simulink model "Lift_Dragforces"  (R2020a)
settings: Solver=VariableStepAuto  StartTime=0.0  StopTime=6  RelTol=1e-3
model workspace (MAT data in the model file):
  T = Simulink.Parameter
  T.Value = [0; 0; 23.07; 17.74; 13.42; 9.93; 7.08; 4.74; 4.8; 3.17; 1.78; 0.59; -0.44; -1.34; -2.13; -2.83; -3.46; -4.02; -4.52; -4.98; -5.39; -4.77; -5.12; -5.43; -5.73]
  T.DataType = 'auto'
  T.Dimensions = [25 1]
  Tw = Simulink.Parameter
  Tw.Value = [0; 0; 24.07; 18.74; 14.42; 10.93; 8.08; 5.74; 5.8; 4.17; 2.78; 1.59; 0.56; -0.34; -1.13; -1.83; -2.46; -3.02; -3.52; -3.98; -4.39; -3.77; -4.12; -4.43; -4.73]
  Tw.DataType = 'auto'
  Tw.Dimensions = [25 1]
  a = Simulink.Parameter
  a.Value = [0.289798575; 0.30459674; 0.314300855; 0.320590761; 0.324695185; 0.327419595; 0.329266982; 0.330547514; 0.331453787; 0.332107409; 0.3325868; 0.332943702; 0.333213067; 0.333419111; 0.333579107; 0.333705864; 0.333809448; 0.333898539; 0.333981756; 0.334069415; 0.334176808; 0.334332409; 0.334606222; 0.335273105; 0.335273105]
  a.DataType = 'auto'
  a.Dimensions = [25 1]
  ad = Simulink.Parameter
  ad.Value = [1.515241086; 0.637108512; 0.353415361; 0.222386755; 0.151082935; 0.108245808; 0.080683396; 0.062013288; 0.048845254; 0.039248859; 0.032063134; 0.026557986; 0.022256717; 0.018837814; 0.016078029; 0.013817996; 0.011940578; 0.010356505; 0.008993998; 0.007789833; 0.006678523; 0.005571335; 0.004290268; 0.002196383; 0.002196383]
  ad.DataType = 'auto'
  ad.Dimensions = [25 1]
  adp5 = Simulink.Parameter
  adp5.Value = [0; 0; 0.161386935; 0.100936667; 0.068015045; 0.048298399; 0.035668845; 0.027176718; 0.026154004; 0.021248319; 0.017584933; 0.014773712; 0.012576934; 0.010833186; 0.009428602; 0.008287644; 0.007359433; 0.006598956; 0.005984102; 0.005511002; 0.005178535; 0.004044009; 0.004168658; 0.004977863; 0.004977863]
  adp5.DataType = 'auto'
  adp5.Dimensions = [25 1]
  ap5 = Simulink.Parameter
  ap5.Value = [0; 0; 0.197308672; 0.193419158; 0.19060639; 0.188320167; 0.186408424; 0.184780447; 0.18622744; 0.185210871; 0.184412939; 0.183708715; 0.183133563; 0.182715678; 0.182454669; 0.182442554; 0.182866993; 0.183770944; 0.185493747; 0.188781814; 0.194498145; 0.176650898; 0.195168855; 0.240212713; 0.240212713]
  ap5.DataType = 'auto'
  ap5.Dimensions = [25 1]
  c = Simulink.Parameter
  c.Value = [3.65 4.43 4.56 4.36 4.03 3.68 3.35 3.05 2.79 2.56 2.37 2.19 2.04 1.91 1.79 1.68 1.59 1.5 1.43 1.36 1.29 1.24 1.18 1.14 1.09]
  c.DataType = 'auto'
  c.Dimensions = [1 25]
  r = Simulink.Parameter
  r.Value = [1.8; 3.6; 5.4; 7.2; 9; 10.8; 12.6; 14.4; 16.2; 18; 19.8; 21.6; 23.4; 25.2; 27; 28.8; 30.6; 32.4; 34.2; 36; 37.8; 39.6; 41.4; 43.2; 45]
  r.DataType = 'auto'
  r.Dimensions = [25 1]
  wind_speed = [3 5]
libraries: dspsrcs4 x1
settings Model: Creator=Dimple  LastModifiedBy=Dimple
settings SolverCC: AlgebraicLoopSolver=LineSearch

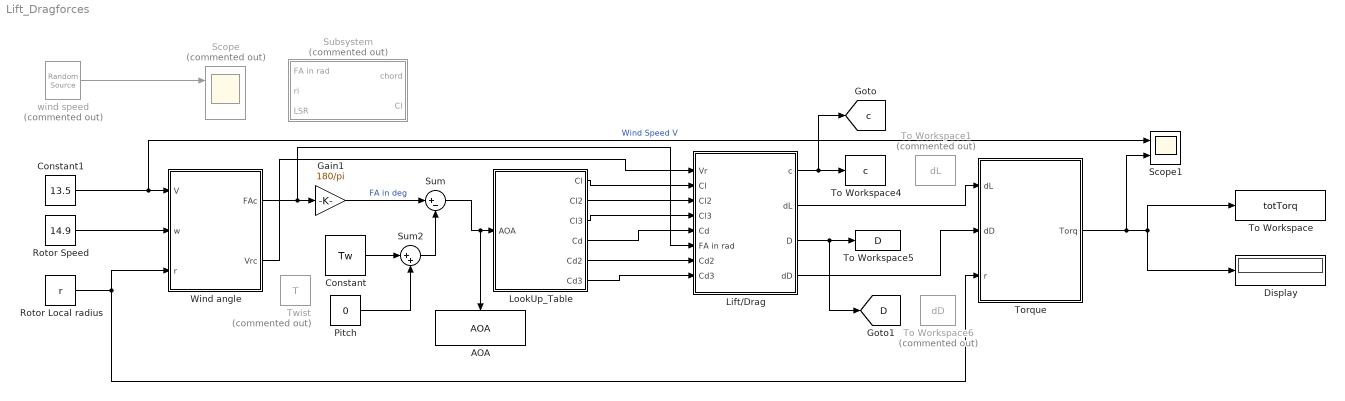
== system Lift_Dragforces ==
  AOA : ToWorkspace  VariableName=AOA  SampleTime=-1
      settings: Save2DSignal=2-D array (concatenate along first dimension)
  Constant : Constant  Value=Tw  VectorParams1D=off  SampleTime=-1
  Constant1 : Constant  Value=13.5
  Display : Display
  Gain1 : Gain  Gain=180/pi
  Lift/Drag : Subsystem
  LookUp_Table : Subsystem
  Pitch : Constant  Value=0
  Rotor Local radius : Constant  Value=r
  Rotor Speed : Constant  Value=14.9  VectorParams1D=off
  Scope : Scope  Commented=on  NumInputPorts=2
  Scope1 : Scope  NumInputPorts=2
  Subsystem : Subsystem  Commented=on
  Sum : Sum  Inputs=|+-
  Sum2 : Sum  Inputs=|++
  To Workspace : ToWorkspace  VariableName=totTorq  SampleTime=-1
      settings: Save2DSignal=2-D array (concatenate along first dimension)
  To Workspace1 : ToWorkspace  Commented=on  VariableName=dL  SampleTime=-1
      settings: Save2DSignal=2-D array (concatenate along first dimension)
  To Workspace4 : ToWorkspace  VariableName=c  SampleTime=-1
      settings: Save2DSignal=2-D array (concatenate along first dimension)
  To Workspace5 : ToWorkspace  VariableName=D  SampleTime=-1
      settings: Save2DSignal=2-D array (concatenate along first dimension)
  To Workspace6 : ToWorkspace  Commented=on  VariableName=dD  SampleTime=-1
      settings: Save2DSignal=2-D array (concatenate along first dimension)
  Torque : Subsystem
  Twist : Constant  Commented=on  Value=T
  Wind angle : Subsystem
  wind speed : dspsrcs4/Random Source  Commented=on  SrcType=Gaussian  NormMethod=Ziggurat  CltLength=12  MinVal=0  MaxVal=1  MeanVal=16  VarVal=2  RepMode=Not repeatable  rawSeed=1  IsInherit=off  SampMode=Discrete  SampTime=1  SampFrame=1  DataType=Double  OutComplex=Real  OutputFrames=off
  tag scope: D=global, c=global
  wires:
  Gain1/1 -> Sum/1  "FA in deg"
  Sum/1 -> AOA/1, LookUp_Table/1(AOA)
  Lift/Drag/2(dL) -> Torque/1(dL)
  Lift/Drag/4(dD) -> Torque/2(dD)
  LookUp_Table/1(Cl) -> Lift/Drag/2(Cl)
  LookUp_Table/2(Cl2) -> Lift/Drag/3(Cl2)
  LookUp_Table/3(Cl3) -> Lift/Drag/4(Cl3)
  LookUp_Table/4(Cd) -> Lift/Drag/5(Cd)
  LookUp_Table/5(Cd2) -> Lift/Drag/7(Cd2)
  LookUp_Table/6(Cd3) -> Lift/Drag/8(Cd3)
  Lift/Drag/1(c) -> [c], To Workspace4/1
  Lift/Drag/3(D) -> [D], To Workspace5/1
  Rotor Local radius/1 -> Torque/3(r), Wind angle/3(r)
  Rotor Speed/1 -> Wind angle/2(w)
  Wind angle/1(FAc) -> Lift/Drag/6(FA in rad), Gain1/1
  Wind angle/2(Vrc) -> Lift/Drag/1(Vr)
  Sum2/1 -> Sum/2
  Pitch/1 -> Sum2/2
  wind speed/1 -> Scope/1
  Constant1/1 -> Scope1/1, Wind angle/1(V)  "Wind Speed V"
  Constant/1 -> Sum2/1
  Torque/1(Torq) -> Display/1, To Workspace/1, Scope1/2

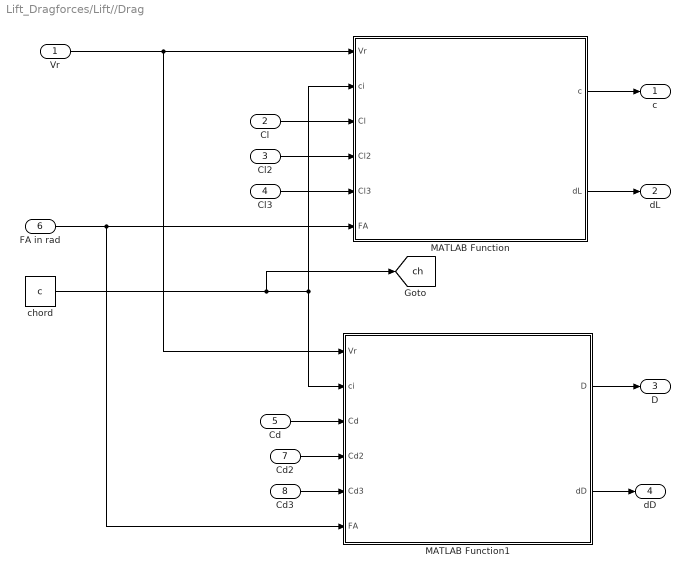
== system Lift_Dragforces/Lift//Drag ==
  Vr : Inport
  Cl : Inport  Port=2
  Cl2 : Inport  Port=3
  Cl3 : Inport  Port=4
  Cd : Inport  Port=5
  FA in rad : Inport  Port=6
  Cd2 : Inport  Port=7
  Cd3 : Inport  Port=8
  MATLAB Function : MATLAB Function  TreatAsAtomicUnit=on
  MATLAB Function1 : MATLAB Function  TreatAsAtomicUnit=on
  chord : Constant  Value=c
  c : Outport
  dL : Outport  Port=2
  D : Outport  Port=3
  dD : Outport  Port=4
  tag scope: ch=global
  wires:
  Cl2/1 -> MATLAB Function/4(Cl2)
  Cl/1 -> MATLAB Function/3(Cl)
  FA in rad/1 -> MATLAB Function1/6(FA), MATLAB Function/6(FA)
  Cd3/1 -> MATLAB Function1/5(Cd3)
  chord/1 -> [ch], MATLAB Function1/2(ci), MATLAB Function/2(ci)
  MATLAB Function/2(dL) -> dL/1
  Vr/1 -> MATLAB Function1/1(Vr), MATLAB Function/1(Vr)
  Cd2/1 -> MATLAB Function1/4(Cd2)
  Cl3/1 -> MATLAB Function/5(Cl3)
  Cd/1 -> MATLAB Function1/3(Cd)
  MATLAB Function1/2(dD) -> dD/1
  MATLAB Function1/1(D) -> D/1
  MATLAB Function/1(c) -> c/1

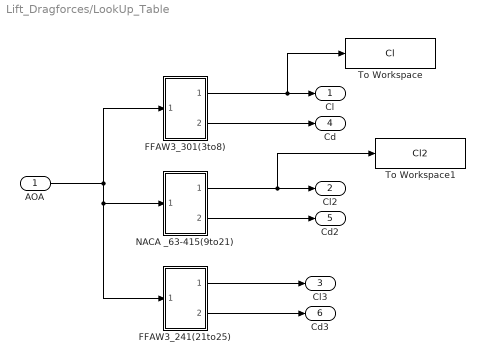
== system Lift_Dragforces/LookUp_Table ==
  AOA : Inport
  FFAW3_241(21to25) : Subsystem
  FFAW3_301(3to8) : Subsystem
  NACA _63-415(9to21) : Subsystem
  To Workspace : ToWorkspace  VariableName=Cl  SampleTime=-1
      settings: Save2DSignal=2-D array (concatenate along first dimension)
  To Workspace1 : ToWorkspace  VariableName=Cl2  SampleTime=-1
      settings: Save2DSignal=2-D array (concatenate along first dimension)
  Cl : Outport
  Cl2 : Outport  Port=2
  Cl3 : Outport  Port=3
  Cd : Outport  Port=4
  Cd2 : Outport  Port=5
  Cd3 : Outport  Port=6
  wires:
  FFAW3_301(3to8)/2(Output1) -> Cd/1
  AOA/1 -> NACA _63-415(9to21)/1(In1), FFAW3_241(21to25)/1(In1), FFAW3_301(3to8)/1(In1)
  FFAW3_301(3to8)/1(Output) -> To Workspace/1, Cl/1
  FFAW3_241(21to25)/1(Output) -> Cl3/1
  FFAW3_241(21to25)/2(Output1) -> Cd3/1
  NACA _63-415(9to21)/2(Output1) -> Cd2/1
  NACA _63-415(9to21)/1(Output) -> To Workspace1/1, Cl2/1

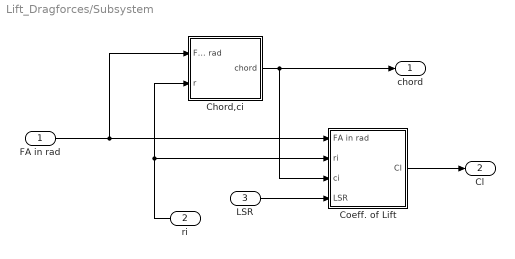
== system Lift_Dragforces/Subsystem ==
  FA in rad : Inport
  ri : Inport  Port=2
  LSR : Inport  Port=3
  Chord,ci : Subsystem
  Coeff. of Lift : Subsystem
  chord : Outport
  Cl : Outport  Port=2
  wires:
  LSR/1 -> Coeff. of Lift/4(LSR)
  FA in rad/1 -> Chord,ci/1(FA in rad), Coeff. of Lift/1(FA in rad)
  ri/1 -> Chord,ci/2(r), Coeff. of Lift/2(ri)
  Coeff. of Lift/1(Cl) -> Cl/1
  Chord,ci/1(chord) -> chord/1, Coeff. of Lift/3(ci)

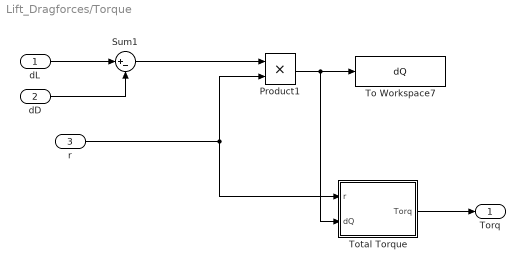
== system Lift_Dragforces/Torque ==
  dL : Inport
  dD : Inport  Port=2
  r : Inport  Port=3
  Product1 : Product
  Sum1 : Sum  Inputs=|+-
  To Workspace7 : ToWorkspace  VariableName=dQ  SampleTime=-1
      settings: Save2DSignal=2-D array (concatenate along first dimension)
  Total Torque : MATLAB Function  TreatAsAtomicUnit=on
  Torq : Outport
  wires:
  r/1 -> Product1/2, Total Torque/1(r)
  Product1/1 -> To Workspace7/1, Total Torque/2(dQ)
  dD/1 -> Sum1/2
  Total Torque/1(Torq) -> Torq/1
  Sum1/1 -> Product1/1
  dL/1 -> Sum1/1

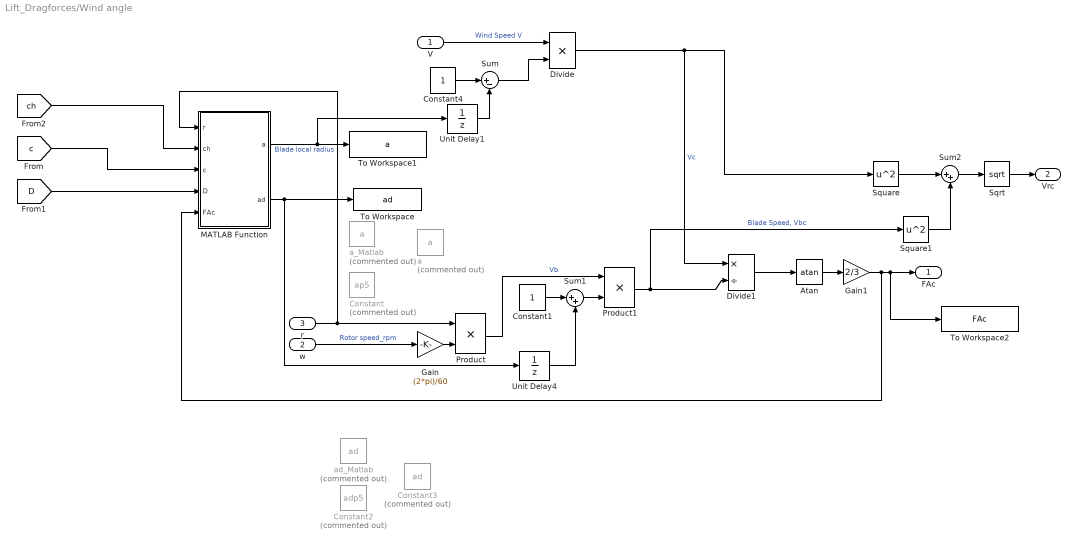
== system Lift_Dragforces/Wind angle ==
  V : Inport
  w : Inport  Port=2
  r : Inport  Port=3
  Atan : Trigonometry  Operator=atan
  Constant : Constant  Commented=on  Value=ap5
  Constant1 : Constant
  Constant2 : Constant  Commented=on  Value=adp5
  Constant3 : Constant  Commented=on  Value=ad
  Constant4 : Constant
  Divide : Product  Inputs=**
  Divide1 : Product  Inputs=*/
  Gain : Gain  Gain=(2*pi)/60
  Gain1 : Gain  Gain=2/3
  MATLAB Function : MATLAB Function  TreatAsAtomicUnit=on
  Product : Product
  Product1 : Product
  Sqrt : Sqrt  SaturateOnIntegerOverflow=on
  Square : Math  Operator=square  SaturateOnIntegerOverflow=on
  Square1 : Math  Operator=square  SaturateOnIntegerOverflow=on
  Sum : Sum  Inputs=|+-
  Sum1 : Sum  Inputs=|++
  Sum2 : Sum  Inputs=|++
  To Workspace : ToWorkspace  VariableName=ad  SampleTime=-1
      settings: Save2DSignal=2-D array (concatenate along first dimension)
  To Workspace1 : ToWorkspace  VariableName=a  SampleTime=-1
      settings: Save2DSignal=2-D array (concatenate along first dimension)
  To Workspace2 : ToWorkspace  VariableName=FAc  SampleTime=-1
      settings: Save2DSignal=2-D array (concatenate along first dimension)
  Unit Delay1 : UnitDelay  SampleTime=-1  HasFrameUpgradeWarning=on
  Unit Delay4 : UnitDelay  SampleTime=-1  HasFrameUpgradeWarning=on
  a : Constant  Commented=on  Value=a
  a_Matlab : Constant  Commented=on  Value=a
  ad_Matlab : Constant  Commented=on  Value=ad
  FAc : Outport
  Vrc : Outport  Port=2
  wires:
  Gain/1 -> Product/2
  Sum/1 -> Divide/2
  Constant4/1 -> Sum/1
  Divide1/1 -> Atan/1
  w/1 -> Gain/1  "Rotor speed_rpm"
  Constant1/1 -> Sum1/1
  Sum1/1 -> Product1/2
  r/1 -> MATLAB Function/1(r), Product/1  "Blade local radius"
  Square/1 -> Sum2/1
  Square1/1 -> Sum2/2
  Sum2/1 -> Sqrt/1
  Sqrt/1 -> Vrc/1
  [ch] -> MATLAB Function/2(ch)
  MATLAB Function/2(ad) -> Unit Delay4/1, To Workspace/1
  MATLAB Function/1(a) -> Unit Delay1/1, To Workspace1/1
  V/1 -> Divide/1  "Wind Speed V"
  Divide/1 -> Divide1/1, Square/1  "Vc"
  Product/1 -> Product1/1  "Vb"
  Product1/1 -> Divide1/2, Square1/1  "Blade Speed, Vbc"
  Atan/1 -> Gain1/1
  Gain1/1 -> MATLAB Function/5(FAc), To Workspace2/1, FAc/1
  Unit Delay1/1 -> Sum/2
  Unit Delay4/1 -> Sum1/2
  [D] -> MATLAB Function/4(D)
  [c] -> MATLAB Function/3(c)

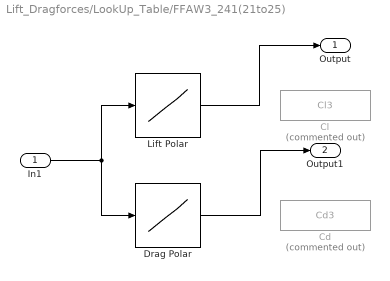
== system Lift_Dragforces/LookUp_Table/FFAW3_241(21to25) ==
  In1 : Inport
  Cd : ToWorkspace  Commented=on  VariableName=Cd3  SampleTime=-1
      settings: Save2DSignal=2-D array (concatenate along first dimension)
  Cl : ToWorkspace  Commented=on  VariableName=Cl3  SampleTime=-1
      settings: Save2DSignal=2-D array (concatenate along first dimension)
  Drag Polar : Lookup_n-D  NumberOfTableDimensions=1  BreakpointsForDimension1=|  Table=|  InternalRulePriority=Speed  RndMeth=Simplest  InputSameDT=on
      BreakpointsForDimension1=|
      | [-4.66442953
      | -3.951342282
      | -3.36409396
      | -2.609060403
      | -1.895973154
      | -1.266778523
      | -0.511744966
      | 0.033557047
      | 0.830536913
      | 1.543624161
      | 2.088926174
      | 2.718120805
      | 3.55704698
      | 4.270134228
      | 5.067114094
      | 6.031879195
      | 6.954697987
      | 7.583892617
      | 8.296979866
      | 8.968120805
      | 9.639261745
      | 10.26845638
      | 11.23322148
      | 11.90436242
      | 12.44966443
      | 12.95302013
      | 13.70805369
      | 14.2533557
      | 14.75671141
      | 15.26006711
      | 15.76342282
      | 16.01510067]
      Table=|
      | [0.010843373
      | 0.010240964
      | 0.009939759
      | 0.010240964
      | 0.009638554
      | 0.009939759
      | 0.009337349
      | 0.009939759
      | 0.009939759
      | 0.010542169
      | 0.010542169
      | 0.011144578
      | 0.011144578
      | 0.011746988
      | 0.012349398
      | 0.012650602
      | 0.014156627
      | 0.014457831
      | 0.014759036
      | 0.016566265
      | 0.017168675
      | 0.017771084
      | 0.020180723
      | 0.021385542
      | 0.022289157
      | 0.023192771
      | 0.026204819
      | 0.028012048
      | 0.031024096
      | 0.034337349
      | 0.039457831
      | 0.041566265]
  Lift Polar : Lookup_n-D  NumberOfTableDimensions=1  BreakpointsForDimension1=|  Table=|  InternalRulePriority=Speed  RndMeth=Simplest  InputSameDT=on
      BreakpointsForDimension1=|
      | [0.165837479
      | 0.870646766
      | 1.451077944
      | 2.031509121
      | 2.529021559
      | 3.109452736
      | 3.565505804
      | 4.104477612
      | 4.60199005
      | 5.016583748
      | 5.679933665
      | 6.343283582
      | 6.92371476
      | 7.587064677
      | 8.084577114
      | 8.830845771
      | 9.577114428
      | 9.950248756
      | 10.61359867
      | 11.35986733
      | 12.10613599
      | 12.89386401
      | 13.64013267
      | 14.51077944
      | 15.46434494
      | 16.12769486
      | 16.83250415
      | 17.66169154
      | 18.44941957
      | 19.32006633
      | 20.02487562
      | 20.77114428
      | 21.51741294
      | 22.30514096
      | 22.96849088
      | 23.79767828
      | 24.25373134
      | 24.66832504]
      Table=|
      | [0.238095238
      | 0.285714286
      | 0.357142857
      | 0.416666667
      | 0.5
      | 0.55952381
      | 0.607142857
      | 0.654761905
      | 0.720238095
      | 0.785714286
      | 0.845238095
      | 0.922619048
      | 1
      | 1.035714286
      | 1.107142857
      | 1.166666667
      | 1.244047619
      | 1.297619048
      | 1.357142857
      | 1.398809524
      | 1.44047619
      | 1.517857143
      | 1.523809524
      | 1.458333333
      | 1.43452381
      | 1.422619048
      | 1.416666667
      | 1.410714286
      | 1.392857143
      | 1.380952381
      | 1.357142857
      | 1.345238095
      | 1.30952381
      | 1.297619048
      | 1.279761905
      | 1.279761905
      | 1.261904762
      | 1.214285714]
  Output : Outport
  Output1 : Outport  Port=2
  wires:
  In1/1 -> Drag Polar/1, Lift Polar/1
  Drag Polar/1 -> Output1/1
  Lift Polar/1 -> Output/1

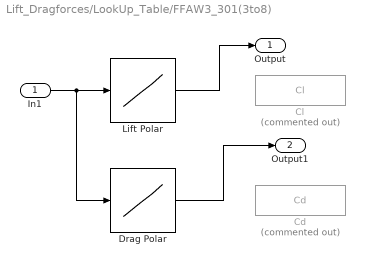
== system Lift_Dragforces/LookUp_Table/FFAW3_301(3to8) ==
  In1 : Inport
  Cd : ToWorkspace  Commented=on  VariableName=Cd  SampleTime=-1
      settings: Save2DSignal=2-D array (concatenate along first dimension)
  Cl : ToWorkspace  Commented=on  VariableName=Cl  SampleTime=-1
      settings: Save2DSignal=2-D array (concatenate along first dimension)
  Drag Polar : Lookup_n-D  NumberOfTableDimensions=1  BreakpointsForDimension1=|  Table=|  InternalRulePriority=Speed  RndMeth=Simplest  InputSameDT=on
      BreakpointsForDimension1=|
      | [0.095846645
      | 0.623003195
      | 1.150159744
      | 1.629392971
      | 2.156549521
      | 2.68370607
      | 3.21086262
      | 3.785942492
      | 4.217252396
      | 4.600638978
      | 5.079872204
      | 5.702875399
      | 6.42172524
      | 7.284345048
      | 7.955271565
      | 8.722044728
      | 9.440894569
      | 10.25559105
      | 10.97444089
      | 11.59744409
      | 12.22044728
      | 12.65175719
      | 13.22683706
      | 13.84984026
      | 14.47284345
      | 15.14376997
      | 15.67092652
      | 16.24600639
      | 16.77316294
      | 17.20447284
      | 17.73162939
      | 18.25878594
      | 18.78594249
      | 19.60063898
      | 20.51118211
      | 21.27795527
      | 21.85303514
      | 22.57188498
      | 23.09904153
      | 23.67412141
      | 24.34504792
      | 24.82428115
      | 25.44728435
      | 25.87859425
      | 26.45367412
      | 26.8370607
      | 27.50798722]
      Table=|
      | [0.050561798
      | 0.049297753
      | 0.049297753
      | 0.049297753
      | 0.049297753
      | 0.048033708
      | 0.049297753
      | 0.049297753
      | 0.050561798
      | 0.050561798
      | 0.050561798
      | 0.050561798
      | 0.051825843
      | 0.051825843
      | 0.053089888
      | 0.054353933
      | 0.061938202
      | 0.074578652
      | 0.079634831
      | 0.092275281
      | 0.094803371
      | 0.097331461
      | 0.10238764
      | 0.1125
      | 0.118820225
      | 0.131460674
      | 0.136516854
      | 0.149157303
      | 0.160533708
      | 0.168117978
      | 0.173174157
      | 0.180758427
      | 0.188342697
      | 0.198455056
      | 0.208567416
      | 0.211095506
      | 0.213623596
      | 0.218679775
      | 0.223735955
      | 0.228792135
      | 0.23258427
      | 0.238904494
      | 0.243960674
      | 0.247752809
      | 0.249016854
      | 0.252808989
      | 0.256601124]
  Lift Polar : Lookup_n-D  NumberOfTableDimensions=1  BreakpointsForDimension1=|  Table=|  InternalRulePriority=Speed  RndMeth=Simplest  InputSameDT=on
      BreakpointsForDimension1=|
      | [0.142857143
      | 0.571428571
      | 1.047619048
      | 1.428571429
      | 1.80952381
      | 2.238095238
      | 2.571428571
      | 2.904761905
      | 3.238095238
      | 3.666666667
      | 4.095238095
      | 4.333333333
      | 4.714285714
      | 5.142857143
      | 5.428571429
      | 5.904761905
      | 6.380952381
      | 6.80952381
      | 7.285714286
      | 7.714285714
      | 8.238095238
      | 8.761904762
      | 9.238095238
      | 10.04761905
      | 10.66666667
      | 11.23809524
      | 11.80952381
      | 12.23809524
      | 12.85714286
      | 13.23809524
      | 13.95238095
      | 14.61904762
      | 15.19047619
      | 15.71428571
      | 16.52380952
      | 17.04761905
      | 17.71428571
      | 18.28571429
      | 18.80952381
      | 19.38095238
      | 19.9047619
      | 20.57142857
      | 21.04761905
      | 21.66666667
      | 22.0952381
      | 22.57142857
      | 23.04761905
      | 23.80952381
      | 24.33333333
      | 25.14285714
      | 25.9047619
      | 26.33333333
      | 26.95238095
      | 27.33333333
      | 27.71428571]
      Table=|
      | [0.175722543
      | 0.249710983
      | 0.295953757
      | 0.351445087
      | 0.411560694
      | 0.467052023
      | 0.499421965
      | 0.54566474
      | 0.587283237
      | 0.638150289
      | 0.684393064
      | 0.726011561
      | 0.767630058
      | 0.804624277
      | 0.860115607
      | 0.897109827
      | 0.952601156
      | 0.989595376
      | 1.031213873
      | 1.07283237
      | 1.114450867
      | 1.146820809
      | 1.165317919
      | 1.165317919
      | 1.151445087
      | 1.156069364
      | 1.183815029
      | 1.211560694
      | 1.230057803
      | 1.267052023
      | 1.280924855
      | 1.299421965
      | 1.304046243
      | 1.313294798
      | 1.304046243
      | 1.29017341
      | 1.271676301
      | 1.253179191
      | 1.225433526
      | 1.202312139
      | 1.179190751
      | 1.165317919
      | 1.165317919
      | 1.156069364
      | 1.132947977
      | 1.132947977
      | 1.119075145
      | 1.058959538
      | 1.049710983
      | 1.01734104
      | 0.989595376
      | 0.975722543
      | 0.952601156
      | 0.929479769
      | 0.906358382]
  Output : Outport
  Output1 : Outport  Port=2
  wires:
  In1/1 -> Drag Polar/1, Lift Polar/1
  Drag Polar/1 -> Output1/1
  Lift Polar/1 -> Output/1

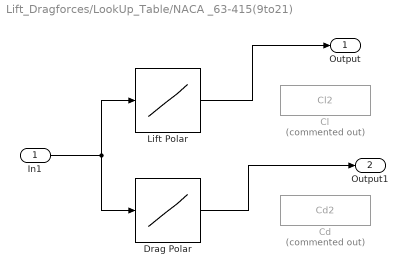
== system Lift_Dragforces/LookUp_Table/NACA _63-415(9to21) ==
  In1 : Inport
  Cd : ToWorkspace  Commented=on  VariableName=Cd2  SampleTime=-1
      settings: Save2DSignal=2-D array (concatenate along first dimension)
  Cl : ToWorkspace  Commented=on  VariableName=Cl2  SampleTime=-1
      settings: Save2DSignal=2-D array (concatenate along first dimension)
  Drag Polar : Lookup_n-D  NumberOfTableDimensions=1  BreakpointsForDimension1=|  Table=|  InternalRulePriority=Speed  RndMeth=Simplest  InputSameDT=on
      BreakpointsForDimension1=|
      | [0.032626427
      | 0.619902121
      | 1.305057096
      | 1.76182708
      | 2.251223491
      | 2.740619902
      | 3.099510604
      | 3.654159869
      | 4.208809135
      | 4.730831974
      | 5.187601958
      | 5.709624796
      | 6.427406199
      | 6.982055465
      | 7.569331158
      | 8.156606852
      | 8.646003263
      | 9.037520392
      | 9.657422512
      | 9.983686786
      | 10.57096248
      | 10.99510604
      | 11.45187602
      | 11.87601958
      | 12.30016313
      | 12.62642741
      | 13.01794454
      | 13.37683524]
      Table=|
      | [0.004635762
      | 0.005099338
      | 0.004635762
      | 0.004635762
      | 0.005099338
      | 0.004635762
      | 0.005562914
      | 0.005562914
      | 0.005562914
      | 0.007417219
      | 0.008344371
      | 0.008344371
      | 0.009735099
      | 0.011125828
      | 0.011125828
      | 0.01205298
      | 0.013907285
      | 0.014834437
      | 0.015298013
      | 0.014834437
      | 0.016225166
      | 0.020860927
      | 0.023178808
      | 0.026887417
      | 0.031523179
      | 0.037086093
      | 0.03986755
      | 0.047284768]
  Lift Polar : Lookup_n-D  NumberOfTableDimensions=1  BreakpointsForDimension1=|  Table=|  InternalRulePriority=Speed  RndMeth=Simplest  InputSameDT=on
      BreakpointsForDimension1=|
      | [0.093603744
      | 0.468018721
      | 0.904836193
      | 1.341653666
      | 1.684867395
      | 2.152886115
      | 2.55850234
      | 3.088923557
      | 3.556942278
      | 4.149765991
      | 4.586583463
      | 4.898595944
      | 5.335413417
      | 5.772230889
      | 6.115444618
      | 6.458658346
      | 6.833073323
      | 7.238689548
      | 7.613104524
      | 7.925117005
      | 8.361934477
      | 8.767550702
      | 9.110764431
      | 9.516380655
      | 9.953198128
      | 10.35881435
      | 10.76443058
      | 11.07644306
      | 11.45085803
      | 12.0124805
      | 12.51170047
      | 12.94851794
      | 13.32293292
      | 13.75975039
      | 14.25897036
      | 14.60218409
      | 14.97659906
      | 15.38221529
      | 15.75663027
      | 16.00624025
      | 16.16224649]
      Table=|
      | [0.369230769
      | 0.432692308
      | 0.473076923
      | 0.530769231
      | 0.576923077
      | 0.623076923
      | 0.657692308
      | 0.709615385
      | 0.773076923
      | 0.807692308
      | 0.876923077
      | 0.923076923
      | 0.963461538
      | 0.992307692
      | 1.009615385
      | 1.05
      | 1.090384615
      | 1.125
      | 1.165384615
      | 1.2
      | 1.246153846
      | 1.280769231
      | 1.309615385
      | 1.35
      | 1.373076923
      | 1.407692308
      | 1.436538462
      | 1.465384615
      | 1.476923077
      | 1.5
      | 1.528846154
      | 1.546153846
      | 1.557692308
      | 1.546153846
      | 1.546153846
      | 1.523076923
      | 1.5
      | 1.482692308
      | 1.476923077
      | 1.459615385
      | 1.442307692]
  Output : Outport
  Output1 : Outport  Port=2
  wires:
  Lift Polar/1 -> Output/1
  Drag Polar/1 -> Output1/1
  In1/1 -> Lift Polar/1, Drag Polar/1

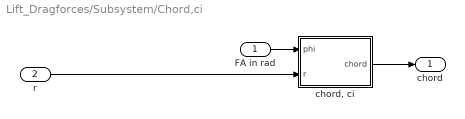
== system Lift_Dragforces/Subsystem/Chord,ci ==
  FA in rad : Inport
  r : Inport  Port=2
  "chord, ci" : MATLAB Function  TreatAsAtomicUnit=on
  chord : Outport
  wires:
  FA in rad/1 -> "chord, ci"/1(phi)
  r/1 -> "chord, ci"/2(r)
  "chord, ci"/1(chord) -> chord/1

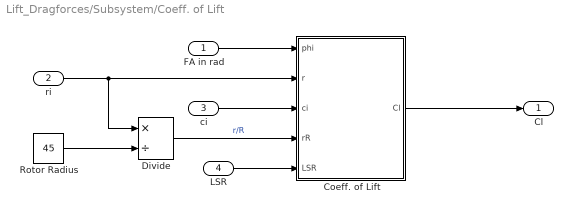
== system Lift_Dragforces/Subsystem/Coeff. of Lift ==
  FA in rad : Inport
  ri : Inport  Port=2
  ci : Inport  Port=3
  LSR : Inport  Port=4
  Coeff. of Lift : MATLAB Function  TreatAsAtomicUnit=on
  Divide : Product  Inputs=*/
  Rotor Radius : Constant  Value=45
  Cl : Outport
  wires:
  ci/1 -> Coeff. of Lift/3(ci)
  LSR/1 -> Coeff. of Lift/5(LSR)
  ri/1 -> Divide/1, Coeff. of Lift/2(r)
  Divide/1 -> Coeff. of Lift/4(rR)  "r/R"
  FA in rad/1 -> Coeff. of Lift/1(phi)
  Rotor Radius/1 -> Divide/2
  Coeff. of Lift/1(Cl) -> Cl/1

== matlab function Lift_Dragforces/Subsystem/Coeff. of Lift/Coeff. of Lift ==
  data: phi input; r input; Cl output; ci input; rR input; LSR input
function Cl = fcn(phi, r, ci, rR, LSR)
B  = 3;                                                                    %No. of Blades
sigma = (B.*ci)./(2*pi()*r);                                               %solidity ratio
F     = (2.*[acos(exp(-[(B/2).*(1-rR)]./[rR.*sin(phi)]))])./pi();          %F 
N     = [4.*F.*sin(phi)].*[cos(phi)-(LSR.*sin(phi))];                      %Numerator
D     = sigma.*[sin(phi)+(LSR.*cos(phi))];                                 %Denominator
Cl    = N./D;                                                              %Coeff. of Lift
end

== matlab function Lift_Dragforces/Subsystem/Chord,ci/chord, ci ==
  data: phi input; chord output; r input
function chord = fcn(phi,r)
%chord, ci = (8*pi()*ri)*(1-cos(phi))/(B*Cldesign)
B  = 3;      %No. of Blades
Cl = 1.3;    %Cldesign
k  = (8*pi())/(B*Cl);
chord = k.* r.*(1-cos(phi));
end

== matlab function Lift_Dragforces/Lift//Drag/MATLAB Function ==
  data: c output; Vr input; ci input; Cl input; Cl2 input; Cl3 input; dL output; FA input
function [c,dL]  = fcn(Vr,ci,Cl, Cl2, Cl3,FA)
% dL  = B*0.5*rho*Vr^2*ci*Cl
B   = 3;                                  %No. of Blades
rho = 1.2;                                %density of air in kg/m3
k   = B*0.5*rho;
c=zeros(25,1);
for i= 1:length(Cl)
    if i>=3 && i<9
        c(i,1)=Cl(i,1);
    elseif i>=9 && i<22
        c(i,1)=Cl2(i,1);
    elseif i>=22
        c(i,1)=Cl3(i,1);
    end
    %fprintf('i=%f c=%f',i,c)
dL  = k.*Vr.*Vr.*ci.*c.*sin(FA) ; 
end

== matlab function Lift_Dragforces/Lift//Drag/MATLAB Function1 ==
  data: D output; Vr input; ci input; Cd input; Cd2 input; Cd3 input; dD output; FA input
function [D,dD]   = fcn(Vr,ci,Cd,Cd2,Cd3,FA)
% dD  = B*0.5*rho*Vr^2*ci*Cd
B   = 3;                                  %No. of Blades
rho = 1.2;                                %density of air in kg/m3
k   = B*0.5*rho;
D=zeros(25,1);
for i= 1:length(Cd)
    if i>=3 && i<9
        D(i,1)=Cd(i,1);
    elseif i>=9 && i<22
        D(i,1)=Cd2(i,1);
    elseif i>=22
        D(i,1)=Cd3(i,1);
    end
    %fprintf('i=%f c=%f',i,c)
dD  = k.*Vr.*Vr.*ci.*D.*cos(FA); 
end

== matlab function Lift_Dragforces/Torque/Total Torque ==
  data: r input; dQ input; Torq output
function Torq = fcn(r, dQ)

Torq = trapz(r,dQ);
end

== matlab function Lift_Dragforces/Wind angle/MATLAB Function ==
  data: a output; r input; ch input; c input; D input; FAc input; ad output
function [a,ad]  = fcn(r,ch,c,D,FAc)
B = 3;                          % No. of Blades
R = 45;                         % Rotor Radius
s = (B.*ch)./(2.*pi.*r);
Cn = (c.*cos(FAc))+(D.*sin(FAc));
Ct = (c.*sin(FAc))-(D.*cos(FAc));
F  = (2/pi)*acos((exp(-((B/2).*(1-(r./R)))./((r./R).*sin(FAc)))));
%z  = exp(-((B/2).*(1-(r./R)))./((r./R).*sin(FAc));
% Axial Induction Factor

a = 1./((4.*F.*sin(FAc).*sin(FAc))./(s.*Cn)+1);
a(1) = 0.21952;
a(2) = 0.21952;
a(25) = a(24);

% Tangential Induction Factor

ad = 1./((4.*F.*sin(FAc).*cos(FAc))./(s.*Ct)-1);
ad(1) = 0.17397;
ad(2) = 0.17397;
ad(25) = ad(24);

end
